simulink model "sampleModel1964"  (R2023a)
settings: Solver=VariableStepAuto  StartTime=0.0  StopTime=10.0  RelTol=1e-3
libraries: hdlsllib x6, simulink x2
settings Model: Creator=user1  LastModifiedBy=user1

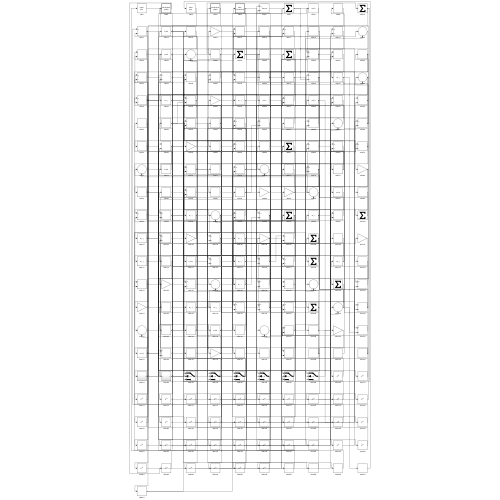
[thumbnail: Simulink's stored preview of the top-level diagram]
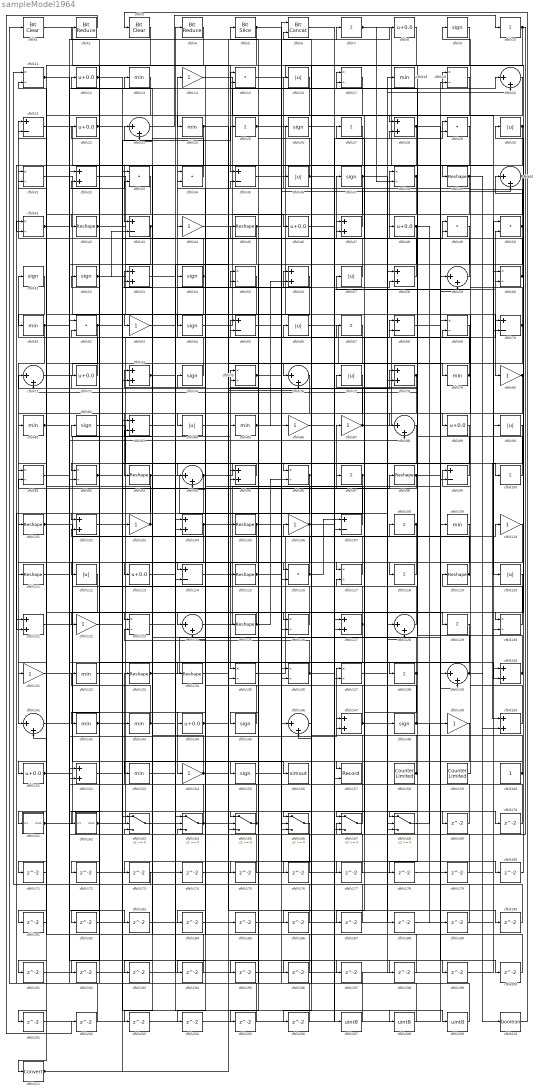
== system sampleModel1964 ==
  cfblk1 : simulink/Logic and Bit Operations/Bit Clear  iBit=0
      settings: LibrarySourceBlock=|
      | hdlsllib/Logic and Bit
      | Operations/Bit Clear
  cfblk{7,10,25,27,67,97,100,108,118,129,138} (11 alike) : Sum  Inputs=+
  cfblk{39,42,45,93,98,101,105,111,115,119,125,133..134} (13 alike) : Reshape
  cfblk{28,32,47,53,56,58,73,78,83,95,102,104,121,127,140,147,150,152} (18 alike) : Sum
  cfblk{14,44,63,80,86..87,103,106,110,122,131,149,154} (13 alike) : Gain
  cfblk{21,35,43,65,68,70,99,107,114} (9 alike) : Sum  Inputs=+-
  cfblk{13,18,24,61,79,81,85,109,132,142..143,153} (12 alike) : MinMax
  cfblk{11,17,19,31,38,41,55,60,69,75,91..92,96,117,123,126,130,135..137} (20 alike) : Product  Inputs=*/  RndMeth=Zero  SaturateOnIntegerOverflow=on
  cfblk{16,30,36,57,66,77,84,90,112,120} (10 alike) : Abs  SaturateOnIntegerOverflow=off
  cfblk{8,12,22,46,48,72,89,113,144,151} (10 alike) : Bias  Bias=0.0  SaturateOnIntegerOverflow=off
  cfblk{15,29,33..34,49..50,62,116} (8 alike) : DotProduct  OutDataTypeStr=Inherit: Inherit via internal rule
  cfblk{20,23,40,59,71,76,88,94,124,128,139,141,146} (13 alike) : Sum  Inputs=|++
  cfblk{9,26,37,51..52,54,64,74,82,145,148,155} (12 alike) : Signum
  cfblk156 : ToWorkspace  VariableName=simout  SaveFormat=Timeseries  SampleTime=-1
  cfblk157 : Record  FileSettingsInternal="{\"entries\":[{\"content\":{\"excelSettings\":{\"content\":{},\"type\":\"Streamout.ExcelSettings\"}},\"type\":\"Streamout.FileSettingStorage\",\"uuid\":\"\"}],\"packageUris\":[\"http:\\/\\/schema.mathworks.com\\/mf0\\/streamout_blocks\\/R2020a\"],\"version\":\"1.0\"}"  Layout=[1 1]  SignalsInternal="{\"entries\":[{\"content\":{\"signals\":[{\"content\":{\"blockPath\":[],\"dimensions\":[1],\"domain\":\"\",\"lineColor\":\"#a2142f\",\"plots\":[1],\"port\":1,\"signalID\":5500,\"signalName\":\"XY Graph:1\"},\"type\":\"RecordBlkView.Signal\",\"uuid\":\"\"},{\"content\":{\"blockPath\":[],\"dimensions\":[1],\"domain\":\"\",\"lineColor\":\"#139fff\",\"plots\":[1],\"port\":2,\"signalID\":5503,\"signalName\":\"XY Graph:2\"},\"type\":\"RecordBlkView.Signal\",\"uuid\":\"\"}]},\"type\":\"RecordBlkView.InputSignals\",\"uuid\":\"\"}],\"packageUris\":[\"http:\\/\\/schema.mathworks.com\\/mf0\\/streamout_blocks\\/R2020a\"],\"version\":\"1.0\"}"  VisualizationBindings="{\"xyplotplugin\":{\"info\":[{\"series\":[{\"bindingParametersList\":[{\"parameter\":\"X-Axis\",\"signalID\":5500,\"signalName\":\"XY Graph:1\"},{\"parameter\":\"Y-Axis\",\"signalID\":5503,\"signalName\":\"XY Graph:2\"}],\"seriesID\":14815}],\"subplotID\":1}]}}"  CompatibilityTag=XY  st=-1
  cfblk158 : hdlsllib/Sources/Counter Limited  uplimit=7  tsamp=-1
  cfblk159 : hdlsllib/Sources/Counter Limited  uplimit=7  tsamp=-1
  cfblk160 : Constant  SampleTime=-1
  cfblk161 : Subsystem
      settings: LibrarySourceBlock=|
      | hdlsllib/Ports &
      | Subsystems/Subsystem
  cfblk162 : Subsystem
      settings: LibrarySourceBlock=|
      | hdlsllib/Ports &
      | Subsystems/Subsystem
  cfblk{163..168} (6 alike) : Switch  SaturateOnIntegerOverflow=off  InputSameDT=off
  cfblk{169..206} (38 alike) : Delay  SampleTime=1
  cfblk2 : hdlsllib/Logic and Bit Operations/Bit Reduce  mode=AND
  cfblk207 : DataTypeConversion  OutDataTypeStr=uint8  SaturateOnIntegerOverflow=off  RndMeth=Floor
  cfblk208 : DataTypeConversion  OutDataTypeStr=uint8  SaturateOnIntegerOverflow=off  RndMeth=Floor
  cfblk209 : DataTypeConversion  OutDataTypeStr=uint8  SaturateOnIntegerOverflow=off  RndMeth=Floor
  cfblk210 : DataTypeConversion  OutDataTypeStr=boolean  SaturateOnIntegerOverflow=off  RndMeth=Floor
  cfblk211 : DataTypeConversion  SaturateOnIntegerOverflow=off  RndMeth=Floor
  cfblk3 : simulink/Logic and Bit Operations/Bit Clear  iBit=0
      settings: LibrarySourceBlock=|
      | hdlsllib/Logic and Bit
      | Operations/Bit Clear
  cfblk4 : hdlsllib/Logic and Bit Operations/Bit Reduce  mode=AND
  cfblk5 : hdlsllib/Logic and Bit Operations/Bit Slice  lidx=7  ridx=0
  cfblk6 : hdlsllib/Logic and Bit Operations/Bit Concat  numInputs=2
  wires:
  cfblk101/1 -> cfblk155/1, cfblk168/3
  cfblk107/1 -> cfblk87/1
  cfblk119/1 -> cfblk75/1, cfblk49/2
  cfblk64/1 -> cfblk19/1
  cfblk168/1 -> cfblk149/1
  cfblk79/1 -> cfblk14/1, cfblk15/2
  cfblk25/1 -> cfblk89/1, cfblk78/2
  cfblk54/1 -> cfblk21/1, cfblk201/1
  cfblk15/1 -> cfblk130/1
  cfblk70/1 -> cfblk34/1, cfblk135/2
  cfblk90/1 -> cfblk150/1
  cfblk31/1 -> cfblk63/1
  cfblk131/1 -> cfblk106/1
  cfblk154/1 -> cfblk108/1, cfblk53/2
  cfblk151/1 -> cfblk85/1, cfblk17/1
  cfblk32/1 -> cfblk148/1
  cfblk135/1 -> cfblk69/1
  cfblk118/1 -> cfblk112/1
  cfblk7/1 -> cfblk39/1, cfblk38/2
  cfblk58/1 -> cfblk37/1
  cfblk11/1 -> cfblk151/1, cfblk88/2
  cfblk108/1 -> cfblk135/1, cfblk102/2
  cfblk167/1 -> cfblk54/1
  cfblk23/1 -> cfblk10/1
  cfblk69/1 -> cfblk117/1
  cfblk27/1 -> cfblk43/1
  cfblk162/1(Out1) -> cfblk4/1, cfblk98/1, cfblk208/1
  cfblk86/1 -> cfblk29/1
  cfblk50/1 -> cfblk9/1, cfblk114/2
  cfblk94/1 -> cfblk100/1, cfblk121/2, cfblk104/2
  cfblk44/1 -> cfblk46/1
  cfblk130/1 -> cfblk119/1
  cfblk164/1 -> cfblk133/1, cfblk76/2
  cfblk53/1 -> cfblk79/1
  cfblk36/1 -> cfblk5/1, cfblk28/2, cfblk176/1
  cfblk9/1 -> cfblk126/1
  cfblk30/1 -> cfblk124/1, cfblk203/1
  cfblk126/1 -> cfblk82/1
  cfblk59/1 -> cfblk27/1
  cfblk34/1 -> cfblk12/1
  cfblk103/1 -> cfblk11/2, cfblk52/1
  cfblk84/1 -> cfblk66/1
  cfblk159/1 -> cfblk69/2
  cfblk106/1 -> cfblk73/1, cfblk125/1, cfblk180/1, cfblk181/1
  cfblk72/1 -> cfblk51/1
  cfblk123/1 -> cfblk156/1
  cfblk96/1 -> cfblk193/1, cfblk194/1
  cfblk19/1 -> cfblk167/1
  cfblk132/1 -> cfblk68/1
  cfblk1/1 -> cfblk35/1
  cfblk21/1 -> cfblk120/1
  cfblk145/1 -> cfblk74/1
  cfblk35/1 -> cfblk16/1
  cfblk148/1 -> cfblk26/1, cfblk70/1
  cfblk42/1 -> cfblk33/1, cfblk105/1
  cfblk8/1 -> cfblk84/1
  cfblk161/1(Out1) -> cfblk95/1, cfblk147/2
  cfblk60/1 -> cfblk30/1, cfblk38/1
  cfblk160/1 -> cfblk153/1, cfblk147/1
  cfblk138/1 -> cfblk23/1, cfblk157/1
  cfblk116/1 -> cfblk13/1, cfblk107/1
  cfblk128/1 -> cfblk44/1
  cfblk104/1 -> cfblk142/1, cfblk190/1
  cfblk12/1 -> cfblk127/2, cfblk116/2, cfblk166/3
  cfblk57/1 -> cfblk2/1
  cfblk81/1 -> cfblk197/1, cfblk198/1
  cfblk158/1 -> cfblk137/1, cfblk67/1
  cfblk140/1 -> cfblk99/1, cfblk71/2
  cfblk95/1 -> cfblk92/1
  cfblk48/1 -> cfblk137/2, cfblk189/1
  cfblk143/1 -> cfblk22/1, cfblk65/2
  cfblk121/1 -> cfblk154/1
  cfblk20/1 -> cfblk24/1
  cfblk83/1 -> cfblk104/1
  cfblk97/1 -> cfblk95/2, cfblk146/2
  cfblk47/1 -> cfblk36/1
  cfblk22/1 -> cfblk162/1(In1), cfblk115/1
  cfblk133/1 -> cfblk109/1, cfblk140/2
  cfblk43/1 -> cfblk92/2, cfblk23/2
  cfblk61/1 -> cfblk141/1, cfblk136/2
  cfblk16/1 -> cfblk163/2
  cfblk10/1 -> cfblk167/2, cfblk28/1
  cfblk63/1 -> cfblk164/2
  cfblk117/1 -> cfblk55/1
  cfblk87/1 -> cfblk50/2, cfblk71/1
  cfblk52/1 -> cfblk146/1, cfblk80/1, cfblk43/2
  cfblk13/1 -> cfblk91/1
  cfblk76/1 -> cfblk114/1
  cfblk85/1 -> cfblk86/1, cfblk56/2
  cfblk134/1 -> cfblk110/1
  cfblk18/1 -> cfblk168/1
  cfblk80/1 -> cfblk93/1, cfblk88/1
  cfblk67/1 -> cfblk167/3
  cfblk3/1 -> cfblk211/1
  cfblk114/1 -> cfblk18/1
  cfblk100/1 -> cfblk77/1
  cfblk122/1 -> cfblk143/1
  cfblk40/1 -> cfblk131/1, cfblk81/1
  cfblk125/1 -> cfblk122/1, cfblk96/2
  cfblk55/1 -> cfblk64/1
  cfblk120/1 -> cfblk145/1
  cfblk56/1 -> cfblk73/2
  cfblk98/1 -> cfblk20/1, cfblk91/2
  cfblk71/1 -> cfblk76/1
  cfblk152/1 -> cfblk165/1
  cfblk41/1 -> cfblk7/1, cfblk166/2, cfblk183/1
  cfblk74/1 -> cfblk31/1
  cfblk136/1 -> cfblk60/2, cfblk123/2
  cfblk75/1 -> cfblk49/1, cfblk47/1
  cfblk65/1 -> cfblk129/1
  cfblk127/1 -> cfblk62/2, cfblk157/2
  cfblk77/1 -> cfblk166/1
  cfblk139/1 -> cfblk72/1, cfblk150/2, cfblk45/1
  cfblk109/1 -> cfblk113/1
  cfblk142/1 -> cfblk25/1, cfblk48/1
  cfblk73/1 -> cfblk68/2, cfblk209/1
  cfblk92/1 -> cfblk65/1, cfblk94/1
  cfblk115/1 -> cfblk17/2, cfblk195/1
  cfblk51/1 -> cfblk61/1
  cfblk153/1 -> cfblk97/1
  cfblk28/1 -> cfblk134/1, cfblk200/1
  cfblk38/1 -> cfblk118/1, cfblk192/1
  cfblk110/1 -> cfblk144/1
  cfblk165/1 -> cfblk32/2, cfblk53/1
  cfblk5/1 -> cfblk101/1, cfblk40/2
  cfblk14/1 -> cfblk90/1
  cfblk105/1 -> cfblk168/2, cfblk184/1
  cfblk99/1 -> cfblk15/1
  cfblk144/1 -> cfblk78/1, cfblk8/1
  cfblk24/1 -> cfblk41/2, cfblk96/1
  cfblk37/1 -> cfblk152/2, cfblk70/2
  cfblk78/1 -> cfblk111/1, cfblk187/1
  cfblk163/1 -> cfblk58/2
  cfblk45/1 -> cfblk138/1, cfblk204/1
  cfblk147/1 -> cfblk20/2, cfblk124/2
  cfblk62/1 -> cfblk103/1, cfblk47/2, cfblk161/1(In1)
  cfblk124/1 -> cfblk59/1
  cfblk102/1 -> cfblk56/1
  cfblk141/1 -> cfblk33/2
  cfblk66/1 -> cfblk128/1
  cfblk93/1 -> cfblk128/2, cfblk102/1
  cfblk39/1 -> cfblk42/1, cfblk210/1
  cfblk82/1 -> cfblk139/2
  cfblk29/1 -> cfblk116/1
  cfblk150/1 -> cfblk57/1
  cfblk111/1 -> cfblk123/1
  cfblk26/1 -> cfblk169/1
  cfblk169/1 -> cfblk32/1
  cfblk91/1 -> cfblk170/1
  cfblk170/1 -> cfblk127/1
  cfblk33/1 -> cfblk171/1
  cfblk171/1 -> cfblk141/2
  cfblk129/1 -> cfblk172/1
  cfblk172/1 -> cfblk60/1
  cfblk166/1 -> cfblk173/1
  cfblk173/1 -> cfblk11/1
  cfblk113/1 -> cfblk174/1
  cfblk174/1 -> cfblk126/2
  cfblk49/1 -> cfblk175/1
  cfblk175/1 -> cfblk163/1
  cfblk176/1 -> cfblk62/1
  cfblk155/1 -> cfblk177/1
  cfblk177/1 -> cfblk165/2
  cfblk149/1 -> cfblk178/1
  cfblk178/1 -> cfblk99/2
  cfblk68/1 -> cfblk179/1
  cfblk179/1 -> cfblk117/2
  cfblk180/1 -> cfblk40/1
  cfblk181/1 -> cfblk31/2
  cfblk4/1 -> cfblk182/1
  cfblk182/1 -> cfblk19/2
  cfblk183/1 -> cfblk130/2
  cfblk184/1 -> cfblk34/2
  cfblk185/1 -> cfblk136/1
  cfblk89/1 -> cfblk186/1
  cfblk186/1 -> cfblk41/1
  cfblk187/1 -> cfblk75/2
  cfblk137/1 -> cfblk188/1
  cfblk188/1 -> cfblk140/1
  cfblk189/1 -> cfblk83/2
  cfblk190/1 -> cfblk94/2
  cfblk112/1 -> cfblk191/1
  cfblk191/1 -> cfblk139/1
  cfblk192/1 -> cfblk59/2
  cfblk193/1 -> cfblk164/1
  cfblk194/1 -> cfblk21/2
  cfblk195/1 -> cfblk58/1
  cfblk17/1 -> cfblk196/1
  cfblk196/1 -> cfblk164/3
  cfblk197/1 -> cfblk1/1
  cfblk198/1 -> cfblk163/3
  cfblk46/1 -> cfblk199/1
  cfblk199/1 -> cfblk50/1
  cfblk200/1 -> cfblk55/2
  cfblk201/1 -> cfblk165/3
  cfblk2/1 -> cfblk202/1
  cfblk202/1 -> cfblk121/1
  cfblk203/1 -> cfblk107/2
  cfblk204/1 -> cfblk29/2
  cfblk88/1 -> cfblk205/1
  cfblk205/1 -> cfblk152/1
  cfblk146/1 -> cfblk206/1
  cfblk206/1 -> cfblk35/2
  cfblk6/1 -> cfblk207/1
  cfblk207/1 -> cfblk132/1
  cfblk208/1 -> cfblk6/1
  cfblk209/1 -> cfblk6/2
  cfblk210/1 -> cfblk3/1
  cfblk211/1 -> cfblk185/1, cfblk83/1

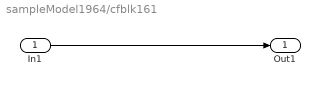
== system sampleModel1964/cfblk161 ==
  In1 : Inport
  Out1 : Outport
  wires:
  In1/1 -> Out1/1

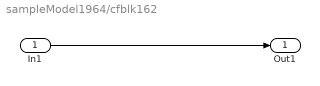
== system sampleModel1964/cfblk162 ==
  In1 : Inport
  Out1 : Outport
  wires:
  In1/1 -> Out1/1
